simulink model "sliding_mode"  (R2021b)
settings: Solver=VariableStepAuto  StartTime=0.0  StopTime=20  FixedStep=0.00001  RelTol=1e-3
libraries: simulink x1
settings Model: Creator=wangchongwei  LastModifiedBy=wangchongwei

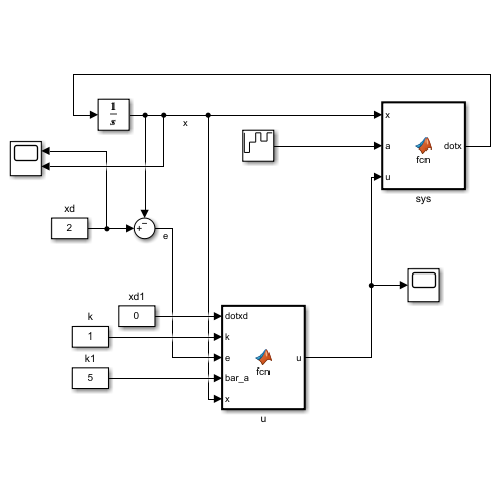
[thumbnail: Simulink's stored preview of the top-level diagram]
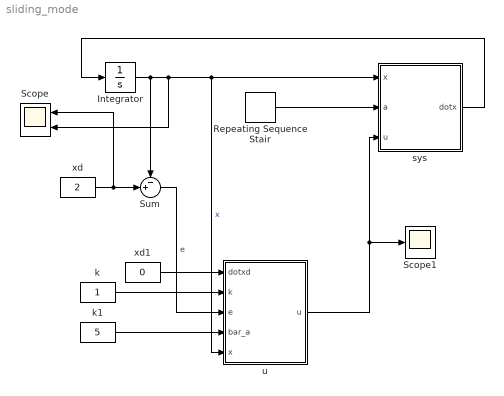
== system sliding_mode ==
  Integrator : Integrator
  Repeating Sequence Stair : simulink/Sources/Repeating Sequence Stair  OutValues=[0.5 0.75 1 0.8 1].'  tsamp=4  OutMin=[]  OutMax=[]  OutDataTypeStr=double  OutputDataTypeScalingMode=double  OutDataType=fixdt(0,8)  ConRadixGroup=Best Precision: Vector-wise  OutScaling=2^-12
  Scope : Scope  NumInputPorts=2
  Scope1 : Scope
  Sum : Sum  Inputs=-+|
  k : Constant
  k1 : Constant  Value=5
  sys : MATLAB Function  TreatAsAtomicUnit=on
  u : MATLAB Function  TreatAsAtomicUnit=on
  xd : Constant  Value=2
  xd1 : Constant  Value=0
  wires:
  Integrator/1 -> Sum/1, Scope/2, u/5(x), sys/1(x)  "x"
  sys/1(dotx) -> Integrator/1
  u/1(u) -> Scope1/1, sys/3(u)
  k/1 -> u/2(k)
  xd/1 -> Scope/1, Sum/2
  Sum/1 -> u/3(e)  "e"
  xd1/1 -> u/1(dotxd)
  Repeating Sequence Stair/1 -> sys/2(a)
  k1/1 -> u/4(bar_a)

== matlab function sliding_mode/sys ==
  data: x input; a input; u input; dotx output
function dotx = fcn(x, a, u)

dotx = a*x^2+u;

== matlab function sliding_mode/u ==
  data: dotxd input; k input; e input; bar_a input; x input; u output
function u = fcn(dotxd, k,e, bar_a, x)

u = dotxd +  k*e+ abs(bar_a) * (x^2+0.1)*(abs(e)/ e);
